simulink model "FlightSimulationOriginal"  (R2021b)
settings: Solver=VariableStepAuto  StartTime=0.0  StopTime=Inf  RelTol=1e-3
undefined symbols (not defined in the file or in its folder): Inertia
libraries: AeroModel x1, AtmosphericModel x1, EoM_6DoF x1, PropulsionModel x1
settings Model: Creator=setup  LastModifiedBy=dmgp1
settings DataIOCC: SaveState=on

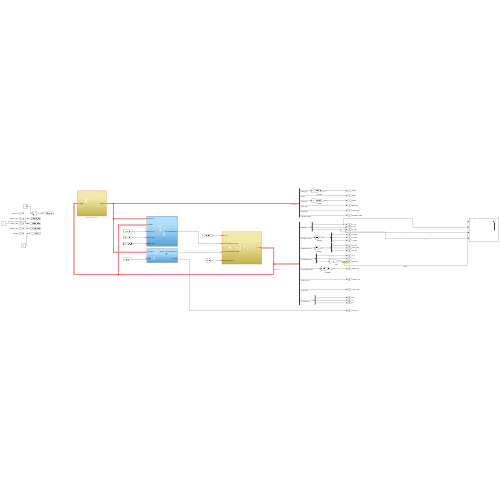
[thumbnail: Simulink's stored preview of the top-level diagram]
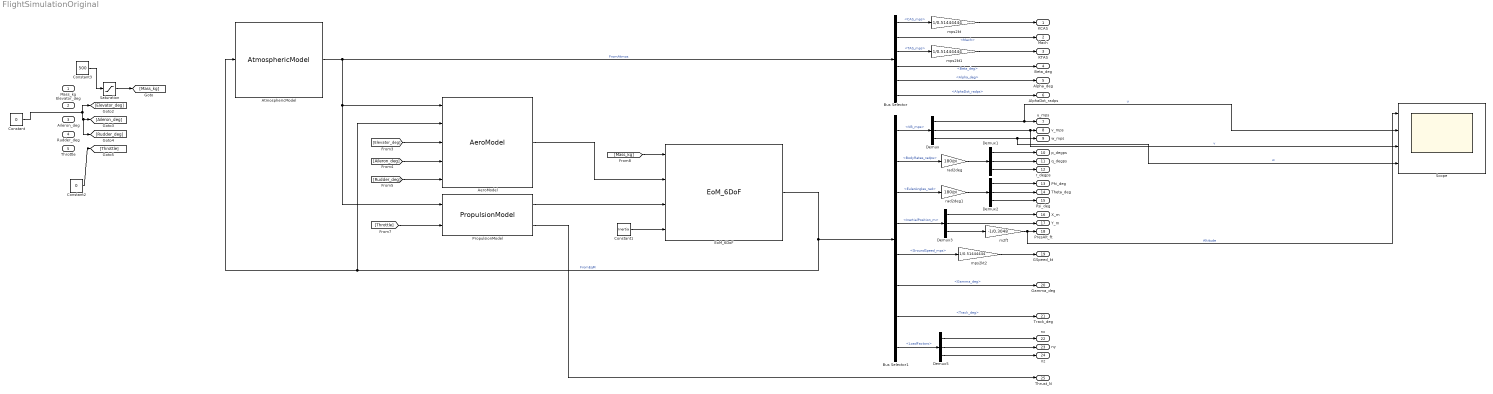
== system FlightSimulationOriginal ==
  Mass_kg : Inport  OutDataTypeStr=double
  Elevator_deg : Inport  Port=2  OutDataTypeStr=double
  Aileron_deg : Inport  Port=3  OutDataTypeStr=double
  Rudder_deg : Inport  Port=4  OutDataTypeStr=double
  Throttle : Inport  Port=5  OutDataTypeStr=double
  AeroModel : AeroModel/AeroModel  SystemSampleTime=-1  VariantActivationTime=update diagram  Latency=0  AutoFrameSizeCalculation=off
  AtmosphericModel : AtmosphericModel/AtmosphericModel  SystemSampleTime=-1  VariantActivationTime=update diagram  Latency=0  AutoFrameSizeCalculation=off
  Bus Selector : BusSelector  OutputSignals=CAS_mps,Mach,TAS_mps,Beta_deg,Alpha_deg,AlphaDot_radps
  Bus Selector1 : BusSelector  OutputSignals=VB_mps,BodyRates_radps,EulerAngles_rad,InertialPosition_m,GroundSpeed_mps,Gamma_deg,Track_deg,LoadFactors
  Constant : Constant  Value=0
  Constant1 : Constant  Value=Inertia  OutDataTypeStr=double
  Constant2 : Constant  Value=0
  Constant3 : Constant  Value=500
  Demux{,1..3,5} (5 alike) : Demux  Outputs=3
  EoM_6DoF : EoM_6DoF/EoM_6DoF  SystemSampleTime=-1  VariantActivationTime=update diagram  Latency=0  AutoFrameSizeCalculation=off
      link override BodyRates/p_radps: InitialCondition=p0
      link override BodyRates/q_radps: InitialCondition=q0
      link override BodyRates/r_radps: InitialCondition=r0
      link override BodyVelocities/u_mps: InitialCondition=u0
      link override BodyVelocities/v_mps: InitialCondition=v0
      link override BodyVelocities/w_mps: InitialCondition=w0
      link override EulerRates/EulerRates/IC: Value=[0 0 0 0 0 0 0 0 0]
      link override EulerRates/PHI_rad: InitialCondition=phi0
      link override EulerRates/PSI_rad: InitialCondition=psi0
      link override EulerRates/THETA_rad: InitialCondition=theta0
      link override InertialData/XI_m: InitialCondition=X0
      link override InertialData/YI_m1: InitialCondition=Y0
      link override InertialData/ZI_m: InitialCondition=Z0
  PropulsionModel : PropulsionModel/PropulsionModel  SystemSampleTime=-1  VariantActivationTime=update diagram  Latency=0  AutoFrameSizeCalculation=off
  Saturation : Saturate  UpperLimit=Inf  LowerLimit=0.1
  Scope : Scope  NumInputPorts=4
  m2ft : Gain  Gain=-1/0.3048
  mps2kt : Gain  Gain=1/0.51444444
  mps2kt1 : Gain  Gain=1/0.51444444
  mps2kt2 : Gain  Gain=1/0.51444444
  rad2deg : Gain  Gain=180/pi
  rad2deg1 : Gain  Gain=180/pi
  KCAS : Outport
  Mach : Outport  Port=2
  KTAS : Outport  Port=3
  Beta_deg : Outport  Port=4
  Alpha_deg : Outport  Port=5
  AlphaDot_radps : Outport  Port=6
  u_mps : Outport  Port=7
  v_mps : Outport  Port=8
  w_mps : Outport  Port=9
  p_degps : Outport  Port=10
  q_degps : Outport  Port=11
  r_degps : Outport  Port=12
  Phi_deg : Outport  Port=13
  Theta_deg : Outport  Port=14
  Psi_deg : Outport  Port=15
  X_m : Outport  Port=16
  Y_m : Outport  Port=17
  PresAlt_ft : Outport  Port=18
  GSpeed_kt : Outport  Port=19
  Gamma_deg : Outport  Port=20
  Track_deg : Outport  Port=21
  nx : Outport  Port=22
  ny : Outport  Port=23
  nz : Outport  Port=24
  Thrust_N : Outport  Port=25
  wires:
  Constant1/1 -> EoM_6DoF/4
  PropulsionModel/1 -> EoM_6DoF/3
  [Mass_kg] -> EoM_6DoF/1
  AeroModel/1 -> EoM_6DoF/2
  PropulsionModel/2 -> Thrust_N/1
  [Aileron_deg] -> AeroModel/4
  [Elevator_deg] -> AeroModel/3
  EoM_6DoF/1 -> AtmosphericModel/1, AeroModel/2, Bus Selector1/1  "FromEqM"
  Demux3/3 -> m2ft/1
  Demux1/2 -> q_degps/1
  Bus Selector1/5 -> mps2kt2/1  "<GroundSpeed_mps>"
  [Rudder_deg] -> AeroModel/5
  Bus Selector/2 -> Mach/1  "<Mach>"
  Bus Selector1/6 -> Gamma_deg/1  "<Gamma_deg>"
  Bus Selector1/4 -> Demux3/1  "<InertialPosition_m>"
  Demux/1 -> Scope/2, u_mps/1  "u"
  Demux2/2 -> Theta_deg/1
  Demux2/1 -> Phi_deg/1
  Demux1/3 -> r_degps/1
  Demux1/1 -> p_degps/1
  Bus Selector/4 -> Beta_deg/1  "<Beta_deg>"
  Bus Selector1/3 -> rad2deg1/1  "<EulerAngles_rad>"
  mps2kt1/1 -> KTAS/1
  Demux/3 -> Scope/4, w_mps/1  "w"
  rad2deg1/1 -> Demux2/1
  Bus Selector/1 -> mps2kt/1  "<CAS_mps>"
  Bus Selector/3 -> mps2kt1/1  "<TAS_mps>"
  Bus Selector/6 -> AlphaDot_radps/1  "<AlphaDot_radps>"
  Bus Selector1/2 -> rad2deg/1  "<BodyRates_radps>"
  Demux/2 -> Scope/3, v_mps/1  "v"
  mps2kt/1 -> KCAS/1
  Demux3/2 -> Y_m/1
  rad2deg/1 -> Demux1/1
  Bus Selector1/8 -> Demux5/1  "<LoadFactors>"
  Bus Selector/5 -> Alpha_deg/1  "<Alpha_deg>"
  Bus Selector1/1 -> Demux/1  "<VB_mps>"
  mps2kt2/1 -> GSpeed_kt/1
  Demux5/2 -> ny/1
  Bus Selector1/7 -> Track_deg/1  "<Track_deg>"
  Demux3/1 -> X_m/1
  Demux5/1 -> nx/1
  Demux2/3 -> Psi_deg/1
  Demux5/3 -> nz/1
  AtmosphericModel/1 -> Bus Selector/1, AeroModel/1, PropulsionModel/1  "FromAtmos"
  [Throttle] -> PropulsionModel/2
  m2ft/1 -> Scope/1, PresAlt_ft/1  "Altitude"
  Saturation/1 -> [Mass_kg]
  Constant3/1 -> Saturation/1
  Constant/1 -> [Elevator_deg], [Rudder_deg], [Aileron_deg]
  Constant2/1 -> [Throttle]
